simulink model "OIRT"  (Simulink 8.5)
settings: Solver=ode3  SolverMode=SingleTasking  StartTime=0.0  StopTime=1.0  FixedStep=2e-5  RelTol=1e-4  AbsTol=1e-6
undefined symbols (not defined in the file or in its folder): DAB, den, elements, num
libraries: powerlib x191, powerlib_extras x6
(part 2 of 9)

== system OIRT/Off-Line Analysis/Line 3 ==
  Fault : Subsystem
  Fault Selector : Subsystem
  Line1 : powerlib/Elements/Distributed Parameters Line  Phases=3  Frequency=ff  Resistance=rr  Inductance=ll  Capacitance=cc  Length=length*faultLocation  x1=[0 -5.51378054187233e-010 123880.156935491 -216580.298623341;3.63428122191995e-005 -5.40254058607506e-010 126835.785979214 -214862.75254025;7.26856244383991e-005 -5.29028650748851e-010 129767.60639827 -213104.874096772;0.000109028436657599 -5.17703937757295e-010 132675.067854194 -211306.993268142;0.000145371248876798 -5.06282045419649e-010 135557.624580994 -209469.447538527;0.000181714061095998 -4.94765117764473e-010 138414.735487598 -207592.581837684]  x2=[0 -3.23724797699364e-010 120565.917523933 -216914.711461437;3.63428122191995e-005 -3.17304179081244e-010 123526.439248582 -215242.540691548;7.26856244383991e-005 -3.10823998596996e-010 126463.773553327 -213529.966270402;0.000109028436657599 -3.04285472655567e-010 129377.369064677 -211777.309669116;0.000145371248876798 -2.97689828618059e-010 132266.678865204 -209984.899882719;0.000181714061095998 -2.91038304567337e-010 135131.160596202 -208153.073368398]  x3=[0 7.44059623378582e-012 410.447611685094 -646.428008619376;3.63428122191995e-005 7.48222855399653e-012 419.265468354708 -640.744004506415;7.26856244383991e-005 7.52245636861023e-012 428.004623780076 -634.939724925513;0.000109028436657599 7.56127212637526e-012 436.663437515089 -629.016259410769;0.000145371248876798 7.59866854110026e-012 445.240284194757 -622.974719868939;0.000181714061095998 7.63463859302189e-012 453.733553840302 -616.816240370712]  x4=[0 -7.74011735582332e-012 481.808085541794 -1056.23567067391;3.63428122191995e-005 -7.77850831267898e-012 496.23380987336 -1049.53553023991;7.26856244383991e-005 -7.81543914861175e-012 510.566385063817 -1042.63837918056;0.000109028436657599 -7.8509029312531e-012 524.803120713916 -1035.54551217527;0.000145371248876798 -7.8848930036183e-012 538.94134441466 -1028.25826064171;0.000181714061095998 -7.91740298535603e-012 552.978402248948 -1020.77799248593]  x5=0.000181714061095998  V1=ones(3,3)  V2=ones(3,3)  I1=ones(3,3)  I2=ones(3,3)  nHarmo=1  Measurements=None
  Line2 : powerlib/Elements/Distributed Parameters Line  Phases=3  Frequency=ff  Resistance=rr  Inductance=ll  Capacitance=cc  Length=length*(1-faultLocation)  x1=[0 -3.23724797699364e-010 120565.917523933 -216914.711461437;3.63428122191995e-005 -3.17304179081244e-010 123526.439248582 -215242.540691548;7.26856244383991e-005 -3.10823998596996e-010 126463.773553327 -213529.966270402;0.000109028436657599 -3.04285472655567e-010 129377.369064677 -211777.309669116;0.000145371248876798 -2.97689828618059e-010 132266.678865204 -209984.899882719;0.000181714061095998 -2.91038304567337e-010 135131.160596202 -208153.073368398]  x2=[0 -3.89220723554692e-011 117247.668058743 -216227.247766345;3.63428122191995e-005 -3.40589983982146e-011 120199.082632705 -214600.6031587;7.26856244383991e-005 -2.91895311513761e-011 123127.934372199 -212933.675399306;0.000109028436657599 -2.43145846733727e-011 126033.673496016 -211226.777390844;0.000145371248876798 -1.94350740511419e-011 128915.754561467 -209480.229538897;0.000181714061095998 -1.45519152283668e-011 131773.63656677 -207694.359691808]  x3=[0 1.32127041726858e-012 461.28727799928 -640.522939590259;3.63428122191995e-005 1.40820533993015e-012 470.019460724035 -634.142961425906;7.26856244383991e-005 1.49487592526663e-012 478.663415060881 -627.643946889944;0.000109028436657599 1.5812659041516e-012 487.217518434115 -621.0271159267;0.000145371248876798 1.66735906013192e-012 495.680165134158 -614.293710596084;0.000181714061095998 1.75313923247169e-012 504.049766618965 -607.444994840437]  x4=[0 -2.15983169985405e-012 405.403824721723 -1059.98981377655;3.63428122191995e-005 -2.24902942782385e-012 419.888153654779 -1054.33609671178;7.26856244383991e-005 -2.33780498552761e-012 434.29366445796 -1048.48446789675;0.000109028436657599 -2.42614170870992e-012 448.617653041113 -1042.43602575358;0.000145371248876798 -2.51402301548996e-012 462.857430616801 -1036.19190564869;0.000181714061095998 -2.60143240947412e-012 477.010324205022 -1029.75327967959]  x5=0.000181714061095998  V1=ones(3,3)  V2=ones(3,3)  I1=ones(3,3)  I2=ones(3,3)  nHarmo=1  Measurements=None
  Timer : powerlib_extras/Control  Blocks/Timer  t=[0 faultTime]  e=[0 1 0 1 0 1]
  A1 : PMIOPort  Tag=PMCPort  Port=1  Side=Left
  B1 : PMIOPort  Tag=PMCPort  Port=2  Side=Left
  C1 : PMIOPort  Tag=PMCPort  Port=3  Side=Left
  A2 : PMIOPort  Tag=PMCPort  Port=4  Side=Right
  B2 : PMIOPort  Tag=PMCPort  Port=5  Side=Right
  C2 : PMIOPort  Tag=PMCPort  Port=6  Side=Right
  wires:
  Fault Selector/1(faultA) -> Fault/1(faultA)
  Fault Selector/2(faultB) -> Fault/2(faultB)
  Fault Selector/3(faultC) -> Fault/3(faultC)
  Fault Selector/4(faultG) -> Fault/4(faultG)
  Timer/1 -> Fault/5(Tfault)
  connections:
  Line1/RConn1 -- Line2/LConn1 -- Fault/LConn1
  Line1/RConn2 -- Line2/LConn2 -- Fault/LConn2
  Line2/LConn3 -- Line1/RConn3 -- Fault/LConn3
  A1/RConn1 -- Line1/LConn1
  B1/RConn1 -- Line1/LConn2
  C1/RConn1 -- Line1/LConn3
  Line2/RConn1 -- A2/RConn1
  Line2/RConn2 -- B2/RConn1
  Line2/RConn3 -- C2/RConn1

== system OIRT/On-Line Analysis/CB-1 ==
  Trip : Inport
  BreakerA : powerlib/Elements/Breaker  InitialState=1  SwitchingTimes="[ 1/60  5/60 ]"  External=on  BreakerResistance=0.01  SnubberResistance=1e6  SnubberCapacitance=inf  Measurements=None  MoreParameters=off  NoBreakLoop=off
  BreakerB : powerlib/Elements/Breaker  InitialState=1  SwitchingTimes="[ 1/60  5/60 ]"  External=on  BreakerResistance=0.01  SnubberResistance=1e6  SnubberCapacitance=inf  Measurements=None  MoreParameters=off  NoBreakLoop=off
  BreakerC : powerlib/Elements/Breaker  InitialState=1  SwitchingTimes="[ 1/60  5/60 ]"  External=on  BreakerResistance=0.01  SnubberResistance=1e6  SnubberCapacitance=inf  Measurements=None  MoreParameters=off  NoBreakLoop=off
  NOT : Logic  Operator=NOT  Inputs=1
  Series RLC Branch1 : powerlib/Elements/Series RLC Branch  LConnTagsString=__new0  RConnTagsString=__new0  BranchType=R  Resistance=1e6  Inductance=1.0  SetiL0=off  InitialCurrent=0  Capacitance=1.0  Setx0=off  InitialVoltage=0  Measurements=None
  Series RLC Branch2 : powerlib/Elements/Series RLC Branch  LConnTagsString=__new0  RConnTagsString=__new0  BranchType=R  Resistance=1e6  Inductance=1.0  SetiL0=off  InitialCurrent=0  Capacitance=1.0  Setx0=off  InitialVoltage=0  Measurements=None
  Series RLC Branch3 : powerlib/Elements/Series RLC Branch  LConnTagsString=__new0  RConnTagsString=__new0  BranchType=R  Resistance=1e6  Inductance=1.0  SetiL0=off  InitialCurrent=0  Capacitance=1.0  Setx0=off  InitialVoltage=0  Measurements=None
  Transport Delay : TransportDelay  DelayTime=t_op+0.001  BufferSize=10240
  A1 : PMIOPort  Tag=PMCPort  Port=1  Side=Left
  B1 : PMIOPort  Tag=PMCPort  Port=2  Side=Left
  C1 : PMIOPort  Tag=PMCPort  Port=3  Side=Left
  A2 : PMIOPort  Tag=PMCPort  Port=4  Side=Right
  B2 : PMIOPort  Tag=PMCPort  Port=5  Side=Right
  C2 : PMIOPort  Tag=PMCPort  Port=6  Side=Right
  wires:
  NOT/1 -> BreakerA/1, BreakerB/1, BreakerC/1
  Transport Delay/1 -> NOT/1
  Trip/1 -> Transport Delay/1
  connections:
  A2/RConn1 -- BreakerA/RConn1 -- Series RLC Branch1/RConn1
  B2/RConn1 -- BreakerB/RConn1 -- Series RLC Branch2/RConn1
  C2/RConn1 -- BreakerC/RConn1 -- Series RLC Branch3/RConn1
  A1/RConn1 -- BreakerA/LConn1 -- Series RLC Branch1/LConn1
  B1/RConn1 -- BreakerB/LConn1 -- Series RLC Branch2/LConn1
  C1/RConn1 -- BreakerC/LConn1 -- Series RLC Branch3/LConn1

== system OIRT/On-Line Analysis/CB-2 ==
  Trip : Inport
  BreakerA : powerlib/Elements/Breaker  InitialState=1  SwitchingTimes="[ 1/60  5/60 ]"  External=on  BreakerResistance=0.01  SnubberResistance=1e6  SnubberCapacitance=inf  Measurements=None  MoreParameters=off  NoBreakLoop=off
  BreakerB : powerlib/Elements/Breaker  InitialState=1  SwitchingTimes="[ 1/60  5/60 ]"  External=on  BreakerResistance=0.01  SnubberResistance=1e6  SnubberCapacitance=inf  Measurements=None  MoreParameters=off  NoBreakLoop=off
  BreakerC : powerlib/Elements/Breaker  InitialState=1  SwitchingTimes="[ 1/60  5/60 ]"  External=on  BreakerResistance=0.01  SnubberResistance=1e6  SnubberCapacitance=inf  Measurements=None  MoreParameters=off  NoBreakLoop=off
  NOT : Logic  Operator=NOT  Inputs=1
  Series RLC Branch1 : powerlib/Elements/Series RLC Branch  LConnTagsString=__new0  RConnTagsString=__new0  BranchType=R  Resistance=1e6  Inductance=1.0  SetiL0=off  InitialCurrent=0  Capacitance=1.0  Setx0=off  InitialVoltage=0  Measurements=None
  Series RLC Branch2 : powerlib/Elements/Series RLC Branch  LConnTagsString=__new0  RConnTagsString=__new0  BranchType=R  Resistance=1e6  Inductance=1.0  SetiL0=off  InitialCurrent=0  Capacitance=1.0  Setx0=off  InitialVoltage=0  Measurements=None
  Series RLC Branch3 : powerlib/Elements/Series RLC Branch  LConnTagsString=__new0  RConnTagsString=__new0  BranchType=R  Resistance=1e6  Inductance=1.0  SetiL0=off  InitialCurrent=0  Capacitance=1.0  Setx0=off  InitialVoltage=0  Measurements=None
  Transport Delay : TransportDelay  DelayTime=t_op+0.001  BufferSize=10240
  A1 : PMIOPort  Tag=PMCPort  Port=1  Side=Left
  B1 : PMIOPort  Tag=PMCPort  Port=2  Side=Left
  C1 : PMIOPort  Tag=PMCPort  Port=3  Side=Left
  A2 : PMIOPort  Tag=PMCPort  Port=4  Side=Right
  B2 : PMIOPort  Tag=PMCPort  Port=5  Side=Right
  C2 : PMIOPort  Tag=PMCPort  Port=6  Side=Right
  wires:
  Trip/1 -> Transport Delay/1
  Transport Delay/1 -> NOT/1
  NOT/1 -> BreakerC/1, BreakerB/1, BreakerA/1
  connections:
  Series RLC Branch3/LConn1 -- BreakerC/LConn1 -- C1/RConn1
  Series RLC Branch2/LConn1 -- BreakerB/LConn1 -- B1/RConn1
  Series RLC Branch1/LConn1 -- BreakerA/LConn1 -- A1/RConn1
  Series RLC Branch3/RConn1 -- BreakerC/RConn1 -- C2/RConn1
  Series RLC Branch2/RConn1 -- BreakerB/RConn1 -- B2/RConn1
  Series RLC Branch1/RConn1 -- BreakerA/RConn1 -- A2/RConn1

== system OIRT/On-Line Analysis/CB-3 ==
  Trip : Inport
  BreakerA : powerlib/Elements/Breaker  InitialState=1  SwitchingTimes="[ 1/60  5/60 ]"  External=on  BreakerResistance=0.01  SnubberResistance=1e6  SnubberCapacitance=inf  Measurements=None  MoreParameters=off  NoBreakLoop=off
  BreakerB : powerlib/Elements/Breaker  InitialState=1  SwitchingTimes="[ 1/60  5/60 ]"  External=on  BreakerResistance=0.01  SnubberResistance=1e6  SnubberCapacitance=inf  Measurements=None  MoreParameters=off  NoBreakLoop=off
  BreakerC : powerlib/Elements/Breaker  InitialState=1  SwitchingTimes="[ 1/60  5/60 ]"  External=on  BreakerResistance=0.01  SnubberResistance=1e6  SnubberCapacitance=inf  Measurements=None  MoreParameters=off  NoBreakLoop=off
  NOT : Logic  Operator=NOT  Inputs=1
  Series RLC Branch1 : powerlib/Elements/Series RLC Branch  LConnTagsString=__new0  RConnTagsString=__new0  BranchType=R  Resistance=1e6  Inductance=1.0  SetiL0=off  InitialCurrent=0  Capacitance=1.0  Setx0=off  InitialVoltage=0  Measurements=None
  Series RLC Branch2 : powerlib/Elements/Series RLC Branch  LConnTagsString=__new0  RConnTagsString=__new0  BranchType=R  Resistance=1e6  Inductance=1.0  SetiL0=off  InitialCurrent=0  Capacitance=1.0  Setx0=off  InitialVoltage=0  Measurements=None
  Series RLC Branch3 : powerlib/Elements/Series RLC Branch  LConnTagsString=__new0  RConnTagsString=__new0  BranchType=R  Resistance=1e6  Inductance=1.0  SetiL0=off  InitialCurrent=0  Capacitance=1.0  Setx0=off  InitialVoltage=0  Measurements=None
  Transport Delay : TransportDelay  DelayTime=t_op+0.001  BufferSize=10240
  A1 : PMIOPort  Tag=PMCPort  Port=1  Side=Left
  B1 : PMIOPort  Tag=PMCPort  Port=2  Side=Left
  C1 : PMIOPort  Tag=PMCPort  Port=3  Side=Left
  A2 : PMIOPort  Tag=PMCPort  Port=4  Side=Right
  B2 : PMIOPort  Tag=PMCPort  Port=5  Side=Right
  C2 : PMIOPort  Tag=PMCPort  Port=6  Side=Right
  wires:
  NOT/1 -> BreakerA/1, BreakerB/1, BreakerC/1
  Transport Delay/1 -> NOT/1
  Trip/1 -> Transport Delay/1
  connections:
  A2/RConn1 -- BreakerA/RConn1 -- Series RLC Branch1/RConn1
  B2/RConn1 -- BreakerB/RConn1 -- Series RLC Branch2/RConn1
  C2/RConn1 -- BreakerC/RConn1 -- Series RLC Branch3/RConn1
  A1/RConn1 -- BreakerA/LConn1 -- Series RLC Branch1/LConn1
  B1/RConn1 -- BreakerB/LConn1 -- Series RLC Branch2/LConn1
  C1/RConn1 -- BreakerC/LConn1 -- Series RLC Branch3/LConn1

== system OIRT/On-Line Analysis/CT&VT-1 ==
  CT-ratio : Gain  Gain=1/CT  SaturateOnIntegerOverflow=on  OutDataTypeStr=Inherit: Same as input  ParamDataTypeStr=Inherit: Same as input
  Ground : powerlib/Elements/Ground  LConnTagsString=a
  IA : powerlib/Measurements/Current Measurement  PhasorSimulation=off  OutputType=Complex  PSBequivalent=0
  IB : powerlib/Measurements/Current Measurement  PhasorSimulation=off  OutputType=Complex  PSBequivalent=0
  IC : powerlib/Measurements/Current Measurement  PhasorSimulation=off  OutputType=Complex  PSBequivalent=0
  Mux : Mux  Inputs=3
  Mux1 : Mux  Inputs=3
  VA : powerlib/Measurements/Voltage Measurement  PhasorSimulation=off  OutputType=Complex  PSBequivalent=0
  VB : powerlib/Measurements/Voltage Measurement  PhasorSimulation=off  OutputType=Complex  PSBequivalent=0
  VC : powerlib/Measurements/Voltage Measurement  PhasorSimulation=off  OutputType=Complex  PSBequivalent=0
  VT-ratio : Gain  Gain=1/VT  SaturateOnIntegerOverflow=on  OutDataTypeStr=Inherit: Same as input  ParamDataTypeStr=Inherit: Same as input
  A1 : PMIOPort  Tag=PMCPort  Port=1  Side=Left
  B1 : PMIOPort  Tag=PMCPort  Port=2  Side=Left
  C1 : PMIOPort  Tag=PMCPort  Port=3  Side=Left
  A2 : PMIOPort  Tag=PMCPort  Port=4  Side=Right
  B2 : PMIOPort  Tag=PMCPort  Port=5  Side=Right
  C2 : PMIOPort  Tag=PMCPort  Port=6  Side=Right
  Vabc : Outport  InitialOutput=0
  Iabc : Outport  Port=2  InitialOutput=0
  wires:
  VC/1 -> Mux1/3
  VB/1 -> Mux1/2
  VA/1 -> Mux1/1
  CT-ratio/1 -> Iabc/1
  Mux/1 -> CT-ratio/1
  VT-ratio/1 -> Vabc/1
  Mux1/1 -> VT-ratio/1
  IA/1 -> Mux/1
  IB/1 -> Mux/2
  IC/1 -> Mux/3
  connections:
  IC/RConn1 -- C2/RConn1
  IB/RConn1 -- B2/RConn1
  A2/RConn1 -- IA/RConn1
  VC/LConn1 -- IC/LConn1 -- C1/RConn1
  VB/LConn1 -- IB/LConn1 -- B1/RConn1
  VA/LConn1 -- IA/LConn1 -- A1/RConn1
  VC/LConn2 -- Ground/LConn1 -- VB/LConn2 -- VA/LConn2

== system OIRT/On-Line Analysis/CT&VT-2 ==
  CT-ratio : Gain  Gain=1/CT  SaturateOnIntegerOverflow=on  OutDataTypeStr=Inherit: Same as input  ParamDataTypeStr=Inherit: Same as input
  Ground : powerlib/Elements/Ground  LConnTagsString=a
  IA : powerlib/Measurements/Current Measurement  PhasorSimulation=off  OutputType=Complex  PSBequivalent=0
  IB : powerlib/Measurements/Current Measurement  PhasorSimulation=off  OutputType=Complex  PSBequivalent=0
  IC : powerlib/Measurements/Current Measurement  PhasorSimulation=off  OutputType=Complex  PSBequivalent=0
  Mux : Mux  Inputs=3
  Mux1 : Mux  Inputs=3
  VA : powerlib/Measurements/Voltage Measurement  PhasorSimulation=off  OutputType=Complex  PSBequivalent=0
  VB : powerlib/Measurements/Voltage Measurement  PhasorSimulation=off  OutputType=Complex  PSBequivalent=0
  VC : powerlib/Measurements/Voltage Measurement  PhasorSimulation=off  OutputType=Complex  PSBequivalent=0
  VT-ratio : Gain  Gain=1/VT  SaturateOnIntegerOverflow=on  OutDataTypeStr=Inherit: Same as input  ParamDataTypeStr=Inherit: Same as input
  A1 : PMIOPort  Tag=PMCPort  Port=1  Side=Left
  B1 : PMIOPort  Tag=PMCPort  Port=2  Side=Left
  C1 : PMIOPort  Tag=PMCPort  Port=3  Side=Left
  A2 : PMIOPort  Tag=PMCPort  Port=4  Side=Right
  B2 : PMIOPort  Tag=PMCPort  Port=5  Side=Right
  C2 : PMIOPort  Tag=PMCPort  Port=6  Side=Right
  Vabc : Outport  InitialOutput=0
  Iabc : Outport  Port=2  InitialOutput=0
  wires:
  IC/1 -> Mux/3
  IB/1 -> Mux/2
  IA/1 -> Mux/1
  Mux1/1 -> VT-ratio/1
  VT-ratio/1 -> Vabc/1
  Mux/1 -> CT-ratio/1
  CT-ratio/1 -> Iabc/1
  VA/1 -> Mux1/1
  VB/1 -> Mux1/2
  VC/1 -> Mux1/3
  connections:
  VA/LConn2 -- VB/LConn2 -- Ground/LConn1 -- VC/LConn2
  A1/RConn1 -- IA/LConn1 -- VA/LConn1
  B1/RConn1 -- IB/LConn1 -- VB/LConn1
  C1/RConn1 -- IC/LConn1 -- VC/LConn1
  A2/RConn1 -- IA/RConn1
  IB/RConn1 -- B2/RConn1
  IC/RConn1 -- C2/RConn1

== system OIRT/On-Line Analysis/CT&VT-3 ==
  CT-ratio : Gain  Gain=1/CT  SaturateOnIntegerOverflow=on  OutDataTypeStr=Inherit: Same as input  ParamDataTypeStr=Inherit: Same as input
  Ground : powerlib/Elements/Ground  LConnTagsString=a
  IA : powerlib/Measurements/Current Measurement  PhasorSimulation=off  OutputType=Complex  PSBequivalent=0
  IB : powerlib/Measurements/Current Measurement  PhasorSimulation=off  OutputType=Complex  PSBequivalent=0
  IC : powerlib/Measurements/Current Measurement  PhasorSimulation=off  OutputType=Complex  PSBequivalent=0
  Mux : Mux  Inputs=3
  Mux1 : Mux  Inputs=3
  VA : powerlib/Measurements/Voltage Measurement  PhasorSimulation=off  OutputType=Complex  PSBequivalent=0
  VB : powerlib/Measurements/Voltage Measurement  PhasorSimulation=off  OutputType=Complex  PSBequivalent=0
  VC : powerlib/Measurements/Voltage Measurement  PhasorSimulation=off  OutputType=Complex  PSBequivalent=0
  VT-ratio : Gain  Gain=1/VT  SaturateOnIntegerOverflow=on  OutDataTypeStr=Inherit: Same as input  ParamDataTypeStr=Inherit: Same as input
  A1 : PMIOPort  Tag=PMCPort  Port=1  Side=Left
  B1 : PMIOPort  Tag=PMCPort  Port=2  Side=Left
  C1 : PMIOPort  Tag=PMCPort  Port=3  Side=Left
  A2 : PMIOPort  Tag=PMCPort  Port=4  Side=Right
  B2 : PMIOPort  Tag=PMCPort  Port=5  Side=Right
  C2 : PMIOPort  Tag=PMCPort  Port=6  Side=Right
  Vabc : Outport  InitialOutput=0
  Iabc : Outport  Port=2  InitialOutput=0
  wires:
  VC/1 -> Mux1/3
  VB/1 -> Mux1/2
  VA/1 -> Mux1/1
  CT-ratio/1 -> Iabc/1
  Mux/1 -> CT-ratio/1
  VT-ratio/1 -> Vabc/1
  Mux1/1 -> VT-ratio/1
  IA/1 -> Mux/1
  IB/1 -> Mux/2
  IC/1 -> Mux/3
  connections:
  IC/RConn1 -- C2/RConn1
  IB/RConn1 -- B2/RConn1
  A2/RConn1 -- IA/RConn1
  VC/LConn1 -- IC/LConn1 -- C1/RConn1
  VB/LConn1 -- IB/LConn1 -- B1/RConn1
  VA/LConn1 -- IA/LConn1 -- A1/RConn1
  VC/LConn2 -- Ground/LConn1 -- VB/LConn2 -- VA/LConn2

== system OIRT/On-Line Analysis/Generator P ==
  Ground : powerlib/Elements/Ground  LConnTagsString=a
  RA : powerlib/Elements/Series RLC Branch  LConnTagsString=__new0  RConnTagsString=__new0  BranchType=RL  Resistance=R  Inductance=L  SetiL0=off  InitialCurrent=0  Capacitance=1.0  Setx0=off  InitialVoltage=0  Measurements=None
  RB : powerlib/Elements/Series RLC Branch  LConnTagsString=__new0  RConnTagsString=__new0  BranchType=RL  Resistance=R  Inductance=L  SetiL0=off  InitialCurrent=0  Capacitance=1.0  Setx0=off  InitialVoltage=0  Measurements=None
  RC : powerlib/Elements/Series RLC Branch  LConnTagsString=__new0  RConnTagsString=__new0  BranchType=RL  Resistance=R  Inductance=L  SetiL0=off  InitialCurrent=0  Capacitance=1.0  Setx0=off  InitialVoltage=0  Measurements=None
  VA : powerlib/Electrical Sources/AC Voltage Source  Amplitude=V  Phase=Phi  Frequency=F  SampleTime=0  Measurements=None
  VB : powerlib/Electrical Sources/AC Voltage Source  Amplitude=V  Phase=Phi-120  Frequency=F  SampleTime=0  Measurements=None
  VC : powerlib/Electrical Sources/AC Voltage Source  Amplitude=V  Phase=Phi+120  Frequency=F  SampleTime=0  Measurements=None
  A : PMIOPort  Tag=PMCPort  Port=1  Side=Right
  B : PMIOPort  Tag=PMCPort  Port=2  Side=Right
  C : PMIOPort  Tag=PMCPort  Port=3  Side=Right
  connections:
  VC/LConn1 -- VA/LConn1 -- Ground/LConn1 -- VB/LConn1
  VA/RConn1 -- RA/LConn1
  VB/RConn1 -- RB/LConn1
  VC/RConn1 -- RC/LConn1
  RA/RConn1 -- A/RConn1
  RB/RConn1 -- B/RConn1
  RC/RConn1 -- C/RConn1

== system OIRT/On-Line Analysis/Generator S ==
  Ground : powerlib/Elements/Ground  LConnTagsString=a
  RA : powerlib/Elements/Series RLC Branch  LConnTagsString=__new0  RConnTagsString=__new0  BranchType=RL  Resistance=R  Inductance=L  SetiL0=off  InitialCurrent=0  Capacitance=1.0  Setx0=off  InitialVoltage=0  Measurements=None
  RB : powerlib/Elements/Series RLC Branch  LConnTagsString=__new0  RConnTagsString=__new0  BranchType=RL  Resistance=R  Inductance=L  SetiL0=off  InitialCurrent=0  Capacitance=1.0  Setx0=off  InitialVoltage=0  Measurements=None
  RC : powerlib/Elements/Series RLC Branch  LConnTagsString=__new0  RConnTagsString=__new0  BranchType=RL  Resistance=R  Inductance=L  SetiL0=off  InitialCurrent=0  Capacitance=1.0  Setx0=off  InitialVoltage=0  Measurements=None
  VA : powerlib/Electrical Sources/AC Voltage Source  Amplitude=V  Phase=Phi  Frequency=F  SampleTime=0  Measurements=Voltage
  VB : powerlib/Electrical Sources/AC Voltage Source  Amplitude=V  Phase=Phi-120  Frequency=F  SampleTime=0  Measurements=Voltage
  VC : powerlib/Electrical Sources/AC Voltage Source  Amplitude=V  Phase=Phi+120  Frequency=F  SampleTime=0  Measurements=None
  A : PMIOPort  Tag=PMCPort  Port=1  Side=Right
  B : PMIOPort  Tag=PMCPort  Port=2  Side=Right
  C : PMIOPort  Tag=PMCPort  Port=3  Side=Right
  connections:
  RC/RConn1 -- C/RConn1
  RB/RConn1 -- B/RConn1
  RA/RConn1 -- A/RConn1
  VC/RConn1 -- RC/LConn1
  VB/RConn1 -- RB/LConn1
  VA/RConn1 -- RA/LConn1
  VB/LConn1 -- Ground/LConn1 -- VA/LConn1 -- VC/LConn1

== system OIRT/On-Line Analysis/Line 1 ==
  Fault : Subsystem
  Fault Selector : Subsystem
  Line1 : powerlib/Elements/Distributed Parameters Line  Phases=3  Frequency=ff  Resistance=rr  Inductance=ll  Capacitance=cc  Length=length*faultLocation  x1=[0 4.11902020198921e-010 134948.186782494 -205850.900154444;3.63428122191995e-005 4.0825381421406e-010 137755.779020702 -203982.723672073;7.26856244383991e-005 4.04528974006798e-010 140537.512818306 -202076.257143491;0.000109028436657599 4.00728198775092e-010 143292.866009928 -200131.858435729;0.000145371248876798 3.96852201970829e-010 146021.321382155 -198149.892536149;0.000181714061095998 3.92901711165905e-010 148722.36677062 -196130.731483934]  x2=[0 7.13787191208823e-010 132490.296601132 -209961.981117024;3.63428122191995e-005 7.1099393994792e-010 135354.443345949 -208127.093081486;7.26856244383991e-005 7.0806722644901e-010 138193.182410169 -206253.13705103;0.000109028436657599 7.05007600091929e-010 141005.98092783 -204340.46479007;0.000145371248876798 7.01815635205876e-010 143792.31090233 -202389.435330525;0.000181714061095998 6.98491930961609e-010 146551.649305534 -200400.414904433]  x3=[0 -6.76275058489345e-013 224.518563642735 -683.917970918056;3.63428122191995e-005 -6.09086881411019e-013 233.867501695858 -680.77776698083;7.26856244383991e-005 -5.41784371293034e-013 243.172539965284 -677.509772749958;0.000109028436657599 -4.74380161637757e-013 252.431931781791 -674.114601667833;0.000145371248876798 -4.068869050378e-013 261.643939044552 -670.592891049494;0.000181714061095998 -3.39317270800973e-013 270.806832547401 -666.945301962996]  x4=[0 3.07147625924859e-012 758.606072926325 -953.210303848756;3.63428122191995e-005 2.97855051235205e-012 771.594320195334 -942.727565252251;7.26856244383991e-005 2.88506565518036e-012 784.437729795524 -932.067865188679;0.000109028436657599 2.7910392359819e-012 797.133890862199 -921.233204613809;0.000145371248876798 2.69648890466286e-012 809.680420171009 -910.225617325636;0.000181714061095998 2.60143240947412e-012 822.074962585311 -899.047169582606]  x5=0.000181714061095998  V1=ones(3,3)  V2=ones(3,3)  I1=ones(3,3)  I2=ones(3,3)  nHarmo=1  Measurements=None
  Line2 : powerlib/Elements/Distributed Parameters Line  Phases=3  Frequency=ff  Resistance=rr  Inductance=ll  Capacitance=cc  Length=length*(1-faultLocation)  x1=[0 7.13787191208823e-010 132490.296601132 -209961.981117024;3.63428122191995e-005 7.1099393994792e-010 135354.443345949 -208127.093081486;7.26856244383991e-005 7.0806722644901e-010 138193.182410169 -206253.13705103;0.000109028436657599 7.05007600091929e-010 141005.98092783 -204340.46479007;0.000145371248876798 7.01815635205876e-010 143792.31090233 -202389.435330525;0.000181714061095998 6.98491930961609e-010 146551.649305534 -200400.414904433]  x2=[0 8.14266724137873e-010 129971.575736346 -213052.577881739;3.63428122191995e-005 8.05963056693762e-010 132878.301564795 -211251.907481799;7.26856244383991e-005 7.97508100149626e-010 135760.084514673 -209411.582521149;0.000109028436657599 7.88903441603976e-010 138616.383640156 -207531.94845124;0.000145371248876798 7.80150696256215e-010 141446.662779046 -205613.358102322;0.000181714061095998 7.71251507103443e-010 144250.390653414 -203656.171617215]  x3=[0 9.9534767771704e-012 277.764627888906 -689.162391337343;3.63428122191995e-005 9.96850032366961e-012 287.180419597183 -685.29219807324;7.26856244383991e-005 9.98165266102339e-012 296.542304036554 -681.293367101691;0.000109028436657599 9.99293132037755e-012 305.848523867077 -677.166649052061;0.000145371248876798 1.00023341845901e-011 315.097332197736 -672.912818559683;0.000181714061095998 1.00098594886287e-011 324.286992914355 -668.532674120445]  x4=[0 -7.55644004758007e-012 685.290952443927 -975.17875177988;3.63428122191995e-005 -7.56361063723915e-012 698.58705925878 -965.698404296413;7.26856244383991e-005 -7.56936144489117e-012 711.752032758518 -956.036783439102;0.000109028436657599 -7.57369139103938e-012 724.783401716979 -946.195702812072;0.000145371248876798 -7.57659966290005e-012 737.678719987202 -936.177009706237;0.000181714061095998 -7.57808571455506e-012 750.435566960599 -925.982584752539]  x5=0.000181714061095998  V1=ones(3,3)  V2=ones(3,3)  I1=ones(3,3)  I2=ones(3,3)  nHarmo=1  Measurements=None
  Timer : powerlib_extras/Control  Blocks/Timer  t=[0 faultTime]  e=[0 1 0 1 0 1]
  A1 : PMIOPort  Tag=PMCPort  Port=1  Side=Left
  B1 : PMIOPort  Tag=PMCPort  Port=2  Side=Left
  C1 : PMIOPort  Tag=PMCPort  Port=3  Side=Left
  A2 : PMIOPort  Tag=PMCPort  Port=4  Side=Right
  B2 : PMIOPort  Tag=PMCPort  Port=5  Side=Right
  C2 : PMIOPort  Tag=PMCPort  Port=6  Side=Right
  wires:
  Timer/1 -> Fault/5(Tfault)
  Fault Selector/4(faultG) -> Fault/4(faultG)
  Fault Selector/3(faultC) -> Fault/3(faultC)
  Fault Selector/2(faultB) -> Fault/2(faultB)
  Fault Selector/1(faultA) -> Fault/1(faultA)
  connections:
  Line2/RConn3 -- C2/RConn1
  Line2/RConn2 -- B2/RConn1
  Line2/RConn1 -- A2/RConn1
  C1/RConn1 -- Line1/LConn3
  B1/RConn1 -- Line1/LConn2
  A1/RConn1 -- Line1/LConn1
  Fault/LConn3 -- Line1/RConn3 -- Line2/LConn3
  Fault/LConn2 -- Line2/LConn2 -- Line1/RConn2
  Fault/LConn1 -- Line2/LConn1 -- Line1/RConn1

== system OIRT/On-Line Analysis/Line 2 ==
  Fault : Subsystem
  Fault Selector : Subsystem
  Line1 : powerlib/Elements/Distributed Parameters Line  Phases=3  Frequency=ff  Resistance=rr  Inductance=ll  Capacitance=cc  Length=length*faultLocation  x1=[0 9.68476217050412e-010 127342.848551577 -214631.49685465;4.36113746630395e-005 9.55734302808782e-010 130854.257052654 -212508.926707786;8.72227493260789e-005 9.42734050039084e-010 134330.295162547 -210328.914609571;0.000130834123989118 9.29478972757876e-010 137770.023295258 -208092.049825363;0.000174445498652158 9.15972653861726e-010 141172.511679509 -205798.936988013;0.000218056873315197 9.02218744158745e-010 144536.840610068 -203450.195934428]  x2=[0 1.36977428205811e-009 123752.137986008 -217168.429652847;4.36113746630395e-005 1.35848190367013e-009 127305.73986734 -215104.549209961;8.72227493260789e-005 1.34682232258328e-009 130824.93053485 -212982.52520933;0.000130834123989118 1.33479869042558e-009 134308.758738242 -210802.931241916;0.000174445498652158 1.32241425722941e-009 137756.282785828 -208566.356460054;0.000218056873315197 1.30967237055302e-009 141166.570799065 -206273.405418207]  x3=[0 8.16545689795399e-013 309.680810749065 -673.085055880316;4.36113746630395e-005 9.02348321687327e-013 320.70471759177 -667.902823103772;8.72227493260789e-005 9.87907045479959e-013 331.641936759414 -662.540053716054;0.000130834123989118 1.07319873433281e-012 342.489511881075 -656.998197293623;0.000174445498652158 1.15820033358593e-012 353.24451081695 -651.278751820831;0.000218056873315197 1.24288886699166e-012 363.904026450925 -645.383263285012]  x4=[0 2.66776398618369e-012 597.298300018826 -1028.19069338857;4.36113746630395e-005 2.55359202678704e-012 614.121399421818 -1018.23193229658;8.72227493260789e-005 2.43872982199108e-012 630.778499531999 -1007.9979393354;0.000130834123989118 2.32320841947591e-012 647.265097873407 -997.491480791277;0.000174445498652158 2.20705904510527e-012 663.57673805734 -986.715396598951;0.000218056873315197 2.09031309448598e-012 679.709010986937 -975.672599573957]  x5=0.000218056873315197  V1=ones(3,3)  V2=ones(3,3)  I1=ones(3,3)  I2=ones(3,3)  nHarmo=1  Measurements=None
  Line2 : powerlib/Elements/Distributed Parameters Line  Phases=3  Frequency=ff  Resistance=rr  Inductance=ll  Capacitance=cc  Length=length*(1-faultLocation)  x1=[0 1.35074945740024e-009 129049.703947902 -214062.823500369;2.90742497753596e-005 1.3428547368374e-009 131388.190834575 -212635.513974521;5.81484995507193e-005 1.33479869042558e-009 133710.893205731 -211182.659165276;8.72227493260789e-005 1.3265822859899e-009 136017.532020069 -209704.433613505;0.000116296999101439 1.3182065106203e-009 138307.830166109 -208201.014908031;0.000145371248876798 1.30967237055302e-009 140581.512495479 -206672.583664294]  x2=[0 1.27469445408267e-009 126664.657270963 -214990.168355112;2.90742497753596e-005 1.27035263845056e-009 129013.451599903 -213588.944463915;5.81484995507193e-005 1.26585820711679e-009 131346.746706153 -212162.060747532;8.72227493260789e-005 1.26121170002655e-009 133664.262275837 -210709.68862676;0.000116296999101439 1.25641367539486e-009 135965.719890779 -209232.00258448;0.000145371248876798 1.25146470963955e-009 138250.84306195 -207729.180144701]  x3=[0 -6.60958513156634e-012 386.932236791552 -661.020303001532;2.90742497753596e-005 -6.62527994219312e-012 394.154117051596 -656.739620291046;5.81484995507193e-005 -6.64017881497047e-012 401.328645021169 -652.380039190519;8.72227493260789e-005 -6.65427996000016e-012 408.454958777694 -647.942083444703;0.000116296999101439 -6.66758168322019e-012 415.53220219088 -643.426286214006;0.000145371248876798 -6.68008238660828e-012 422.559525025574 -638.833190010437]  x4=[0 1.00043707885194e-011 560.464821743637 -1021.34193891781;2.90742497753596e-005 9.99859974711001e-012 571.625588712501 -1015.13760591045;5.81484995507193e-005 9.99162750906445e-012 582.717682591968 -1008.81131783856;8.72227493260789e-005 9.98345491200293e-012 593.739770816856 -1002.36383472014;0.000116296999101439 9.97408293775253e-012 604.690529232223 -995.795931133169;0.000145371248876798 9.9635127122293e-012 615.568642252435 -989.108396122495]  x5=0.000145371248876798  V1=ones(3,3)  V2=ones(3,3)  I1=ones(3,3)  I2=ones(3,3)  nHarmo=1  Measurements=None
  Timer : powerlib_extras/Control  Blocks/Timer  t=[0 faultTime]  e=[0 1 0 1 0 1]
  A1 : PMIOPort  Tag=PMCPort  Port=1  Side=Left
  B1 : PMIOPort  Tag=PMCPort  Port=2  Side=Left
  C1 : PMIOPort  Tag=PMCPort  Port=3  Side=Left
  A2 : PMIOPort  Tag=PMCPort  Port=4  Side=Right
  B2 : PMIOPort  Tag=PMCPort  Port=5  Side=Right
  C2 : PMIOPort  Tag=PMCPort  Port=6  Side=Right
  wires:
  Timer/1 -> Fault/5(Tfault)
  Fault Selector/4(faultG) -> Fault/4(faultG)
  Fault Selector/3(faultC) -> Fault/3(faultC)
  Fault Selector/2(faultB) -> Fault/2(faultB)
  Fault Selector/1(faultA) -> Fault/1(faultA)
  connections:
  Line2/RConn3 -- C2/RConn1
  Line2/RConn2 -- B2/RConn1
  Line2/RConn1 -- A2/RConn1
  C1/RConn1 -- Line1/LConn3
  B1/RConn1 -- Line1/LConn2
  A1/RConn1 -- Line1/LConn1
  Fault/LConn3 -- Line1/RConn3 -- Line2/LConn3
  Fault/LConn2 -- Line2/LConn2 -- Line1/RConn2
  Fault/LConn1 -- Line2/LConn1 -- Line1/RConn1

== system OIRT/On-Line Analysis/Line 3 ==
  Fault : Subsystem
  Fault Selector : Subsystem
  Line1 : powerlib/Elements/Distributed Parameters Line  Phases=3  Frequency=ff  Resistance=rr  Inductance=ll  Capacitance=cc  Length=length*faultLocation  x1=[0 1.26688267164788e-009 124013.51239019 -216527.954508775;3.63428122191995e-005 1.26136003511701e-009 126968.411777735 -214808.586303586;7.26856244383991e-005 1.25560062591656e-009 129899.477645133 -213048.895905675;0.000109028436657599 1.2496055251579e-009 132806.159795557 -211249.213630401;0.000145371248876798 1.24337585819461e-009 135687.912609299 -209409.877300086;0.000181714061095998 1.23691279441118e-009 138544.195146194 -207531.232180603]  x2=[0 1.07566125394806e-009 120673.621416387 -216872.043066564;3.63428122191995e-005 1.0704764059666e-009 123633.548454503 -215198.400705394;7.26856244383991e-005 1.06509061650189e-009 126570.26796701 -213484.362978581;0.000109028436657599 1.05950489653233e-009 129483.228695822 -211730.251631921;0.000145371248876798 1.05372029456571e-009 132371.883842665 -209936.395933519;0.000181714061095998 1.04773789644241e-009 135235.691171723 -208103.132611976]  x3=[0 9.41634785503522e-013 410.201047091308 -644.704764729202;3.63428122191995e-005 8.66710752951941e-013 418.995317618923 -639.024300408645;7.26856244383991e-005 7.9162402821651e-013 427.710937612881 -633.22388342959;0.000109028436657599 7.16388705991664e-013 436.346271044963 -627.304602601078;0.000145371248876798 6.41018908865398e-013 444.899696957714 -621.267569044349;0.000181714061095998 5.65528784668288e-013 453.369609768723 -615.113915984264]  x4=[0 3.49311551261348e-012 482.996612124979 -1057.62072840101;3.63428122191995e-005 3.53101931616844e-012 497.44120087393 -1050.90417457578;7.26856244383991e-005 3.56826030431261e-012 511.792413839749 -1043.99035321395;0.000109028436657599 3.60483148645809e-012 526.047557124648 -1036.88056212415;0.000145371248876798 3.64072599774776e-012 540.203954864294 -1029.57613590092;0.000181714061095998 3.67593710034387e-012 554.258949730096 -1022.0784456742]  x5=0.000181714061095998  V1=ones(3,3)  V2=ones(3,3)  I1=ones(3,3)  I2=ones(3,3)  nHarmo=1  Measurements=None
  Line2 : powerlib/Elements/Distributed Parameters Line  Phases=3  Frequency=ff  Resistance=rr  Inductance=ll  Capacitance=cc  Length=length*(1-faultLocation)  x1=[0 1.07566125394806e-009 120673.621416387 -216872.043066564;3.63428122191995e-005 1.0704764059666e-009 123633.548454503 -215198.400705394;7.26856244383991e-005 1.06509061650189e-009 126570.26796701 -213484.362978581;0.000109028436657599 1.05950489653233e-009 129483.228695822 -211730.251631921;0.000145371248876798 1.05372029456571e-009 132371.883842665 -209936.395933519;0.000181714061095998 1.04773789644241e-009 135235.691171723 -208103.132611976]  x2=[0 5.61138656558577e-010 117329.2471565 -216194.19505847;3.63428122191995e-005 5.59715018090032e-010 120280.201235512 -214566.435879509;7.26856244383991e-005 5.58186314283004e-010 123208.577253105 -212898.399962415;0.000109028436657599 5.56552832093849e-010 126113.825517368 -211190.400417882;0.000145371248876798 5.54814878147107e-010 128995.400677753 -209442.757858267;0.000181714061095998 5.5297277867794e-010 131852.761827442 -207655.800337401]  x3=[0 -4.5112829567783e-012 460.94123695176 -638.804119501438;3.63428122191995e-005 -4.65139768233198e-012 469.649903479229 -632.429043590328;7.26856244383991e-005 -4.79063928378478e-012 478.270410989192 -625.935253030898;0.000109028436657599 -4.92898162378911e-012 486.801141307204 -619.323966786873;0.000145371248876798 -5.0663987337997e-012 495.240493111093 -612.596425877352;0.000181714061095998 -5.20286481894825e-012 503.586882231548 -605.753893143852]  x4=[0 7.66830192130632e-012 406.489639364674 -1061.43877690348;3.63428122191995e-005 7.78895421920646e-012 420.993717890471 -1055.77004765334;7.26856244383991e-005 7.90814443535959e-012 435.418770758496 -1049.90313748285;0.000109028436657599 8.0258501963078e-012 449.762090210312 -1043.83914768265;0.000145371248876798 8.14204940724352e-012 464.020983829842 -1037.57921653759;0.000181714061095998 8.256720256157e-012 478.192775048769 -1031.12451911316]  x5=0.000181714061095998  V1=ones(3,3)  V2=ones(3,3)  I1=ones(3,3)  I2=ones(3,3)  nHarmo=1  Measurements=None
  Timer : powerlib_extras/Control  Blocks/Timer  t=[0 faultTime]  e=[0 1 0 1 0 1]
  A1 : PMIOPort  Tag=PMCPort  Port=1  Side=Left
  B1 : PMIOPort  Tag=PMCPort  Port=2  Side=Left
  C1 : PMIOPort  Tag=PMCPort  Port=3  Side=Left
  A2 : PMIOPort  Tag=PMCPort  Port=4  Side=Right
  B2 : PMIOPort  Tag=PMCPort  Port=5  Side=Right
  C2 : PMIOPort  Tag=PMCPort  Port=6  Side=Right
  wires:
  Fault Selector/1(faultA) -> Fault/1(faultA)
  Fault Selector/2(faultB) -> Fault/2(faultB)
  Fault Selector/3(faultC) -> Fault/3(faultC)
  Fault Selector/4(faultG) -> Fault/4(faultG)
  Timer/1 -> Fault/5(Tfault)
  connections:
  Line1/RConn1 -- Line2/LConn1 -- Fault/LConn1
  Line1/RConn2 -- Line2/LConn2 -- Fault/LConn2
  Line2/LConn3 -- Line1/RConn3 -- Fault/LConn3
  A1/RConn1 -- Line1/LConn1
  B1/RConn1 -- Line1/LConn2
  C1/RConn1 -- Line1/LConn3
  Line2/RConn1 -- A2/RConn1
  Line2/RConn2 -- B2/RConn1
  Line2/RConn3 -- C2/RConn1

== system OIRT/On-Line Analysis/ZR-1 ==
  Vabc : Inport
  Iabc : Inport  Port=2
  Impedance Relay Scheme : Subsystem  mask{fCut=250, fSampling=60*32, WindowSize=10, VoltageRange=110/sqrt(3), CurrentRange=40, ZoneTime=ZoneTime, ZoneImpedance=ZoneImpedance, LineAngle=LineAngle, k0m1=k0m1, k0a1=k0a1, underV=underV}
      mask prompts: fCut "fCut (Hz):"; fSampling "fSampling (Hz):"; WindowSize "Window Size (samples):"; VoltageRange "Voltage Range (V):"; CurrentRange "Current Range (A):"; ZoneTime "Zone Times:"; ZoneImpedance "Zone Impedances:"; LineAngle "Line Angle:"; underV "UnderVoltage Threshold (V):"
  Trip : Outport  InitialOutput=0
  Logic : Outport  Port=2  InitialOutput=0
  FaultType : Outport  Port=3  InitialOutput=0
  FaultZone : Outport  Port=4  InitialOutput=0
  wires:
  Impedance Relay Scheme/4(FaultZone) -> FaultZone/1
  Impedance Relay Scheme/3(FaultType) -> FaultType/1
  Impedance Relay Scheme/2(Logic) -> Logic/1
  Impedance Relay Scheme/1("TRIP ") -> Trip/1
  Vabc/1 -> Impedance Relay Scheme/1(Vabc)
  Iabc/1 -> Impedance Relay Scheme/2(Iabc)

== system OIRT/On-Line Analysis/ZR-2 ==
  Vabc : Inport
  Iabc : Inport  Port=2
  Impedance Relay Scheme : Subsystem  mask{fCut=250, fSampling=60*32, WindowSize=10, VoltageRange=110/sqrt(3), CurrentRange=40, ZoneTime=ZoneTime, ZoneImpedance=ZoneImpedance, LineAngle=LineAngle, k0m1=k0m1, k0a1=k0a1, underV=underV}
      mask prompts: fCut "fCut (Hz):"; fSampling "fSampling (Hz):"; WindowSize "Window Size (samples):"; VoltageRange "Voltage Range (V):"; CurrentRange "Current Range (A):"; ZoneTime "Zone Times:"; ZoneImpedance "Zone Impedances:"; LineAngle "Line Angle:"; underV "UnderVoltage Threshold (V):"
  Trip : Outport  InitialOutput=0
  Logic : Outport  Port=2  InitialOutput=0
  FaultType : Outport  Port=3  InitialOutput=0
  FaultZone : Outport  Port=4  InitialOutput=0
  wires:
  Impedance Relay Scheme/4(FaultZone) -> FaultZone/1
  Impedance Relay Scheme/3(FaultType) -> FaultType/1
  Impedance Relay Scheme/2(Logic) -> Logic/1
  Impedance Relay Scheme/1("TRIP ") -> Trip/1
  Vabc/1 -> Impedance Relay Scheme/1(Vabc)
  Iabc/1 -> Impedance Relay Scheme/2(Iabc)

== system OIRT/On-Line Analysis/ZR-3 ==
  Vabc : Inport
  Iabc : Inport  Port=2
  Impedance Relay Scheme : Subsystem  mask{fCut=250, fSampling=60*32, WindowSize=10, VoltageRange=110/sqrt(3), CurrentRange=40, ZoneTime=ZoneTime, ZoneImpedance=ZoneImpedance, LineAngle=LineAngle, k0m1=k0m1, k0a1=k0a1, underV=underV}
      mask prompts: fCut "fCut (Hz):"; fSampling "fSampling (Hz):"; WindowSize "Window Size (samples):"; VoltageRange "Voltage Range (V):"; CurrentRange "Current Range (A):"; ZoneTime "Zone Times:"; ZoneImpedance "Zone Impedances:"; LineAngle "Line Angle:"; underV "UnderVoltage Threshold (V):"
  Trip : Outport  InitialOutput=0
  Logic : Outport  Port=2  InitialOutput=0
  FaultType : Outport  Port=3  InitialOutput=0
  FaultZone : Outport  Port=4  InitialOutput=0
  wires:
  Iabc/1 -> Impedance Relay Scheme/2(Iabc)
  Vabc/1 -> Impedance Relay Scheme/1(Vabc)
  Impedance Relay Scheme/1("TRIP ") -> Trip/1
  Impedance Relay Scheme/2(Logic) -> Logic/1
  Impedance Relay Scheme/3(FaultType) -> FaultType/1
  Impedance Relay Scheme/4(FaultZone) -> FaultZone/1

== system OIRT/Off-Line Analysis/Line 1/Fault ==
  faultA : Inport
  faultB : Inport  Port=2
  faultC : Inport  Port=3
  faultG : Inport  Port=4
  Tfault : Inport  Port=5
  &{,1..3} (4 alike) : Logic
  BreakerA : powerlib/Elements/Breaker  InitialState=0  SwitchingTimes="[ 1/60  5/60 ]"  External=on  BreakerResistance=0.01  SnubberResistance=1e6  SnubberCapacitance=inf  Measurements=None  MoreParameters=off  NoBreakLoop=off
  BreakerB : powerlib/Elements/Breaker  InitialState=0  SwitchingTimes="[ 1/60  5/60 ]"  External=on  BreakerResistance=0.01  SnubberResistance=1e6  SnubberCapacitance=inf  Measurements=None  MoreParameters=off  NoBreakLoop=off
  BreakerC : powerlib/Elements/Breaker  InitialState=0  SwitchingTimes="[ 1/60  5/60 ]"  External=on  BreakerResistance=0.01  SnubberResistance=1e6  SnubberCapacitance=inf  Measurements=None  MoreParameters=off  NoBreakLoop=off
  BreakerN : powerlib/Elements/Breaker  InitialState=0  SwitchingTimes="[ 1/60  5/60 ]"  External=on  BreakerResistance=0.01  SnubberResistance=1e6  SnubberCapacitance=inf  Measurements=None  MoreParameters=off  NoBreakLoop=off
  Ground : powerlib/Elements/Ground  LConnTagsString=a
  RA : powerlib/Elements/Series RLC Branch  LConnTagsString=__new0  RConnTagsString=__new0  BranchType=R  Resistance=10000  Inductance=1e-3  SetiL0=off  InitialCurrent=0  Capacitance=1e-6  Setx0=off  InitialVoltage=0  Measurements=None
  RB : powerlib/Elements/Series RLC Branch  LConnTagsString=__new0  RConnTagsString=__new0  BranchType=R  Resistance=10000  Inductance=1e-3  SetiL0=off  InitialCurrent=0  Capacitance=1e-6  Setx0=off  InitialVoltage=0  Measurements=None
  RC : powerlib/Elements/Series RLC Branch  LConnTagsString=__new0  RConnTagsString=__new0  BranchType=R  Resistance=10000  Inductance=1e-3  SetiL0=off  InitialCurrent=0  Capacitance=1e-6  Setx0=off  InitialVoltage=0  Measurements=None
  RN : powerlib/Elements/Series RLC Branch  LConnTagsString=__new0  RConnTagsString=__new0  BranchType=R  Resistance=10000  Inductance=1e-3  SetiL0=off  InitialCurrent=0  Capacitance=1e-6  Setx0=off  InitialVoltage=0  Measurements=None
  RfA : powerlib/Elements/Series RLC Branch  LConnTagsString=__new0  RConnTagsString=__new0  BranchType=R  Resistance=faultR  Inductance=1e-3  SetiL0=off  InitialCurrent=0  Capacitance=1e-6  Setx0=off  InitialVoltage=0  Measurements=None
  RfB : powerlib/Elements/Series RLC Branch  LConnTagsString=__new0  RConnTagsString=__new0  BranchType=R  Resistance=faultR  Inductance=1e-3  SetiL0=off  InitialCurrent=0  Capacitance=1e-6  Setx0=off  InitialVoltage=0  Measurements=None
  RfC : powerlib/Elements/Series RLC Branch  LConnTagsString=__new0  RConnTagsString=__new0  BranchType=R  Resistance=faultR  Inductance=1e-3  SetiL0=off  InitialCurrent=0  Capacitance=1e-6  Setx0=off  InitialVoltage=0  Measurements=None
  A : PMIOPort  Tag=PMCPort  Port=1  Side=Left
  B : PMIOPort  Tag=PMCPort  Port=2  Side=Left
  C : PMIOPort  Tag=PMCPort  Port=3  Side=Left
  wires:
  faultA/1 -> &/1
  faultB/1 -> &1/1
  faultC/1 -> &2/1
  faultG/1 -> &3/1
  Tfault/1 -> &3/2, &2/2, &1/2, &/2
  &3/1 -> BreakerN/1
  &/1 -> BreakerA/1
  &1/1 -> BreakerB/1
  &2/1 -> BreakerC/1
  connections:
  B/RConn1 -- RB/LConn1 -- BreakerB/LConn1
  A/RConn1 -- BreakerA/LConn1 -- RA/LConn1
  RC/LConn1 -- C/RConn1 -- BreakerC/LConn1
  BreakerC/RConn1 -- RC/RConn1 -- RfC/LConn1
  RB/RConn1 -- RfB/LConn1 -- BreakerB/RConn1
  RA/RConn1 -- RfA/LConn1 -- BreakerA/RConn1
  BreakerN/LConn1 -- RN/LConn1 -- RfB/RConn1 -- RfA/RConn1 -- RfC/RConn1
  BreakerN/RConn1 -- Ground/LConn1 -- RN/RConn1

== system OIRT/Off-Line Analysis/Line 1/Fault Selector ==
  "  " : Constant  Value=faultType
  "  +" : Logic  Operator=OR  Inputs=7
  " +" : Logic  Operator=OR  Inputs=5
  + : Logic  Operator=OR  Inputs=5
  "+ " : Logic  Operator=OR  Inputs=6
  A-B-C : Fcn  Expr=(u(1)==8)
  A-B-C-G : Fcn  Expr=(u(1)==9)
  A-G : Fcn  Expr=(u(1)==1)
  B-C : Fcn  Expr=(u(1)==4)
  B-C-G : Fcn  Expr=(u(1)==5)
  B-G : Fcn  Expr=(u(1)==2)
  C-A : Fcn  Expr=(u(1)==6)
  C-A-G : Fcn  Expr=(u(1)==7)
  C-G : Fcn  Expr=(u(1)==3)
  faultA : Outport  InitialOutput=0
  faultB : Outport  Port=2  InitialOutput=0
  faultC : Outport  Port=3  InitialOutput=0
  faultG : Outport  Port=4  InitialOutput=0
  wires:
  "  "/1 -> C-G/1, A-G/1, B-G/1, B-C/1, C-A/1, C-A-G/1, A-B-C/1, A-B-C-G/1, B-C-G/1
  +/1 -> faultA/1
  " +"/1 -> faultB/1
  "  +"/1 -> faultC/1
  "+ "/1 -> faultG/1
  A-G/1 -> "+ "/1, +/1
  C-A/1 -> "  +"/4, +/2
  B-G/1 -> " +"/1, "+ "/2
  B-C/1 -> "  +"/2, " +"/2
  B-C-G/1 -> "  +"/3, "+ "/4, " +"/3
  C-G/1 -> "  +"/1, "+ "/3
  C-A-G/1 -> "  +"/5, "+ "/5, +/3
  A-B-C-G/1 -> " +"/5, "  +"/7, "+ "/6, +/5
  A-B-C/1 -> " +"/4, "  +"/6, +/4

== system OIRT/Off-Line Analysis/Line 2/Fault ==
  faultA : Inport
  faultB : Inport  Port=2
  faultC : Inport  Port=3
  faultG : Inport  Port=4
  Tfault : Inport  Port=5
  &{,1..3} (4 alike) : Logic
  BreakerA : powerlib/Elements/Breaker  InitialState=0  SwitchingTimes="[ 1/60  5/60 ]"  External=on  BreakerResistance=0.01  SnubberResistance=1e6  SnubberCapacitance=inf  Measurements=None  MoreParameters=off  NoBreakLoop=off
  BreakerB : powerlib/Elements/Breaker  InitialState=0  SwitchingTimes="[ 1/60  5/60 ]"  External=on  BreakerResistance=0.01  SnubberResistance=1e6  SnubberCapacitance=inf  Measurements=None  MoreParameters=off  NoBreakLoop=off
  BreakerC : powerlib/Elements/Breaker  InitialState=0  SwitchingTimes="[ 1/60  5/60 ]"  External=on  BreakerResistance=0.01  SnubberResistance=1e6  SnubberCapacitance=inf  Measurements=None  MoreParameters=off  NoBreakLoop=off
  BreakerN : powerlib/Elements/Breaker  InitialState=0  SwitchingTimes="[ 1/60  5/60 ]"  External=on  BreakerResistance=0.01  SnubberResistance=1e6  SnubberCapacitance=inf  Measurements=None  MoreParameters=off  NoBreakLoop=off
  Ground : powerlib/Elements/Ground  LConnTagsString=a
  RA : powerlib/Elements/Series RLC Branch  LConnTagsString=__new0  RConnTagsString=__new0  BranchType=R  Resistance=10000  Inductance=1e-3  SetiL0=off  InitialCurrent=0  Capacitance=1e-6  Setx0=off  InitialVoltage=0  Measurements=None
  RB : powerlib/Elements/Series RLC Branch  LConnTagsString=__new0  RConnTagsString=__new0  BranchType=R  Resistance=10000  Inductance=1e-3  SetiL0=off  InitialCurrent=0  Capacitance=1e-6  Setx0=off  InitialVoltage=0  Measurements=None
  RC : powerlib/Elements/Series RLC Branch  LConnTagsString=__new0  RConnTagsString=__new0  BranchType=R  Resistance=10000  Inductance=1e-3  SetiL0=off  InitialCurrent=0  Capacitance=1e-6  Setx0=off  InitialVoltage=0  Measurements=None
  RN : powerlib/Elements/Series RLC Branch  LConnTagsString=__new0  RConnTagsString=__new0  BranchType=R  Resistance=10000  Inductance=1e-3  SetiL0=off  InitialCurrent=0  Capacitance=1e-6  Setx0=off  InitialVoltage=0  Measurements=None
  RfA : powerlib/Elements/Series RLC Branch  LConnTagsString=__new0  RConnTagsString=__new0  BranchType=R  Resistance=faultR  Inductance=1e-3  SetiL0=off  InitialCurrent=0  Capacitance=1e-6  Setx0=off  InitialVoltage=0  Measurements=None
  RfB : powerlib/Elements/Series RLC Branch  LConnTagsString=__new0  RConnTagsString=__new0  BranchType=R  Resistance=faultR  Inductance=1e-3  SetiL0=off  InitialCurrent=0  Capacitance=1e-6  Setx0=off  InitialVoltage=0  Measurements=None
  RfC : powerlib/Elements/Series RLC Branch  LConnTagsString=__new0  RConnTagsString=__new0  BranchType=R  Resistance=faultR  Inductance=1e-3  SetiL0=off  InitialCurrent=0  Capacitance=1e-6  Setx0=off  InitialVoltage=0  Measurements=None
  A : PMIOPort  Tag=PMCPort  Port=1  Side=Left
  B : PMIOPort  Tag=PMCPort  Port=2  Side=Left
  C : PMIOPort  Tag=PMCPort  Port=3  Side=Left
  wires:
  faultA/1 -> &/1
  faultB/1 -> &1/1
  faultC/1 -> &2/1
  faultG/1 -> &3/1
  Tfault/1 -> &3/2, &2/2, &1/2, &/2
  &3/1 -> BreakerN/1
  &/1 -> BreakerA/1
  &1/1 -> BreakerB/1
  &2/1 -> BreakerC/1
  connections:
  B/RConn1 -- RB/LConn1 -- BreakerB/LConn1
  A/RConn1 -- BreakerA/LConn1 -- RA/LConn1
  RC/LConn1 -- C/RConn1 -- BreakerC/LConn1
  BreakerC/RConn1 -- RC/RConn1 -- RfC/LConn1
  RB/RConn1 -- RfB/LConn1 -- BreakerB/RConn1
  RA/RConn1 -- RfA/LConn1 -- BreakerA/RConn1
  BreakerN/LConn1 -- RN/LConn1 -- RfB/RConn1 -- RfA/RConn1 -- RfC/RConn1
  BreakerN/RConn1 -- Ground/LConn1 -- RN/RConn1

== system OIRT/Off-Line Analysis/Line 2/Fault Selector ==
  "  " : Constant  Value=faultType
  "  +" : Logic  Operator=OR  Inputs=7
  " +" : Logic  Operator=OR  Inputs=5
  + : Logic  Operator=OR  Inputs=5
  "+ " : Logic  Operator=OR  Inputs=6
  A-B-C : Fcn  Expr=(u(1)==8)
  A-B-C-G : Fcn  Expr=(u(1)==9)
  A-G : Fcn  Expr=(u(1)==1)
  B-C : Fcn  Expr=(u(1)==4)
  B-C-G : Fcn  Expr=(u(1)==5)
  B-G : Fcn  Expr=(u(1)==2)
  C-A : Fcn  Expr=(u(1)==6)
  C-A-G : Fcn  Expr=(u(1)==7)
  C-G : Fcn  Expr=(u(1)==3)
  faultA : Outport  InitialOutput=0
  faultB : Outport  Port=2  InitialOutput=0
  faultC : Outport  Port=3  InitialOutput=0
  faultG : Outport  Port=4  InitialOutput=0
  wires:
  "  "/1 -> C-G/1, A-G/1, B-G/1, B-C/1, C-A/1, C-A-G/1, A-B-C/1, A-B-C-G/1, B-C-G/1
  +/1 -> faultA/1
  " +"/1 -> faultB/1
  "  +"/1 -> faultC/1
  "+ "/1 -> faultG/1
  A-G/1 -> "+ "/1, +/1
  C-A/1 -> "  +"/4, +/2
  B-G/1 -> " +"/1, "+ "/2
  B-C/1 -> "  +"/2, " +"/2
  B-C-G/1 -> "  +"/3, "+ "/4, " +"/3
  C-G/1 -> "  +"/1, "+ "/3
  C-A-G/1 -> "  +"/5, "+ "/5, +/3
  A-B-C-G/1 -> " +"/5, "  +"/7, "+ "/6, +/5
  A-B-C/1 -> " +"/4, "  +"/6, +/4
